simulink model "analysis_rand6"  (R2017b)
settings: Solver=VariableStepAuto  StartTime=0.0  StopTime=20  RelTol=1e-3
undefined symbols (not defined in the file or in its folder): get
libraries: commsynccomp2 x1, dspspect3 x1, dspsnks4 x1
settings Model: Creator=CQC  LastModifiedBy=CQC

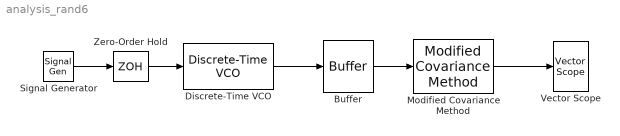
== system analysis_rand6 ==
  Buffer : Buffer  N=1024  OutputFrames=off
  Discrete-Time VCO : commsynccomp2/Discrete-Time VCO  Ac=1  Fc=1500  Kc=1  Ph=0  ts=0.000125
      settings: SourceProductName=Communications System Toolbox  SourceProductBaseCode=CM
  Modified Covariance Method : dspspect3/Modified Covariance Method  ord=6  inheritFFT=off  fftsize=256  inheritTs=on  Ts=1
      settings: SourceProductName=DSP System Toolbox  SourceProductBaseCode=DS
  Signal Generator : SignalGenerator  Units=rad/sec
  Vector Scope : dspsnks4/Vector Scope  ScopeProperties=on  Domain=Frequency  HorizSpan=1  DisplayProperties=off  AxisGrid=on  Memory=off  FrameNumber=on  AxisLegend=off  AxisZoom=off  OpenScopeAtSimStart=on  OpenScopeImmediately=off  FigPos=get(0,'defaultfigureposition')  AxisProperties=off  XUnits=Hertz  XRange=[0...Fs]  InheritXIncr=on  XIncr=1  XLabel=Time  XLimit=Auto  XMin=0  XMax=1  XStart=0  YUnits=dB  YLabel=Amplitude  LineProperties=off  XAxisParamsVer=6.9
      settings: SourceProductName=DSP System Toolbox  SourceProductBaseCode=DS  YMin=-10  YMax=10
  Zero-Order Hold : ZeroOrderHold  SampleTime=8000
  wires:
  Signal Generator/1 -> Zero-Order Hold/1
  Zero-Order Hold/1 -> Discrete-Time VCO/1
  Discrete-Time VCO/1 -> Buffer/1
  Buffer/1 -> Modified Covariance Method/1
  Modified Covariance Method/1 -> Vector Scope/1
